simulink model "RL5_6kg_2021a_enc"  (R2021a)
settings: Solver=ode4  StartTime=0.0  StopTime=time(end)  FixedStep=0.001  RelTol=1e-6
model workspace: external: MATLAB File robot_6kg_v4_EXa5_DataFile.m (data not in the file)
values from neighbouring files (symbols this model uses):
  hI4 = I4wg + I4uch    [RL5_6kg_Dynamic_Param.m]
  hI5 = I5uch + I5ws    [RL5_6kg_Dynamic_Param.m]
  I4g = k4^2*Ig4    [RL5_6kg_Dynamic_Param.m]
  IAB = (Im + IA + IB)    [Basic_3DoF_Delta_Dynamic_Param.m]    (also in RL5_6kg_Dynamic_Param.m)
  lB = l1*(rho1*m1 + me)    [Basic_3DoF_Delta_Dynamic_Param.m]    (also in RL5_6kg_Dynamic_Param.m)
  m4 = 0    [Basic_3DoF_Delta_Dynamic_Param.m]    (also in RL5_6kg_Dynamic_Param.m = Inertias.Solid(10).mass)
  m5 = 0    [Basic_3DoF_Delta_Dynamic_Param.m]    (also in RL5_6kg_Dynamic_Param.m = Inertias.Solid(11).mass)
  m6l = 0    [Basic_3DoF_Delta_Dynamic_Param.m]    (also in RL5_6kg_Dynamic_Param.m = mls_a4 + mls_a5)
  m6u = 0    [Basic_3DoF_Delta_Dynamic_Param.m]    (also in RL5_6kg_Dynamic_Param.m = mus_a4 + mus_a5)
  mD = m3 + 3*m2 + 3*me    [Basic_3DoF_Delta_Dynamic_Param.m]    (also in RL5_6kg_Dynamic_Param.m = m3 + 3*m2 + 3*me + mls_a4_spi + mls_a5_spi + mls_a5_worm)
  rho2 = Sro2    [Basic_3DoF_Delta_Dynamic_Param.m]    (also in RL5_6kg_Dynamic_Param.m)
  rho6l = Sro6l    [RL5_6kg_Dynamic_Param.m]
  rho6u = Sro6u    [RL5_6kg_Dynamic_Param.m]
  tI4 = I4us + I4ls + I4ucr    [RL5_6kg_Dynamic_Param.m]
  tI5 = I5us + I5ls + I5ucr    [RL5_6kg_Dynamic_Param.m]
libraries: eeGeneralControl x5, simulink x5
settings Model: Creator=SUSTRVOJ  LastModifiedBy=alikoc
settings SolverCC: AlgebraicLoopSolver=TrustRegion
settings DataIOCC: SaveOutput=off  SignalLogging=off  DSMLogging=off  SaveTime=off  ReturnWorkspaceOutputs=off
settings DebuggingCC: SFMachineParentedDataDiag=warning
settings DiagnosticsConfigSet: SimMechanicsJointTargetOverSpecification=warning
settings ExplorerConfigSet: InternalSimMechanicsExplorerSettings="<ExplorerConfiguration><canonicalview>default</canonicalview><AnimationSetting><BasePlaybackSpeed>1.0</BasePlaybackSpeed><PlaybackSpeedFactor>1.0</PlaybackSpeedFactor></AnimationSetting><TilePanel><TileInfo><Tiles Columns=\"1\" Count=\"1\" Rows=\"1\"><Column Weight=\"1\"/><Row Weight=\"1\"/><Tile Height=\"1\" Width=\"1\" X=\"0\" Y=\"0\"/></Tiles></TileInfo><SceneInfo><SceneViewer><BGColor><R>0.60000002384185791</R><G>0.60000002384185791</G><B>0.60000002384185791</B></BGColor><Camera><DoPerspective>off</DoPerspective><Position><X>0.135215272225856747</X><Y>-1.20095496527992429</Y><Z>-0.491222676043407747</Z></Position><Center><X>0.135215272225856747</X><Y>5.5511151231257827e-17</Y><Z>-0.491222676043407747</Z></Center><Up><X>0</X><Y>-0</Y><Z>1</Z></Up><ViewLimDist>1</ViewLimDist><YLim>0.916798880077600797</YLim><XLim>1.0012025864974432</XLim></Camera></SceneViewer></SceneInfo></TilePanel><MechEditorPanel><Cameras/><GfxPanelCameraMap/><VideoCreator><PlaybackSpeedRatio>1.0</PlaybackSpeedRatio><FrameRate>30</FrameRate><VideoFormat>Motion JPEG AVI</VideoFormat><FrameSize>auto</FrameSize></VideoCreator></MechEditorPanel></ExplorerConfiguration>"

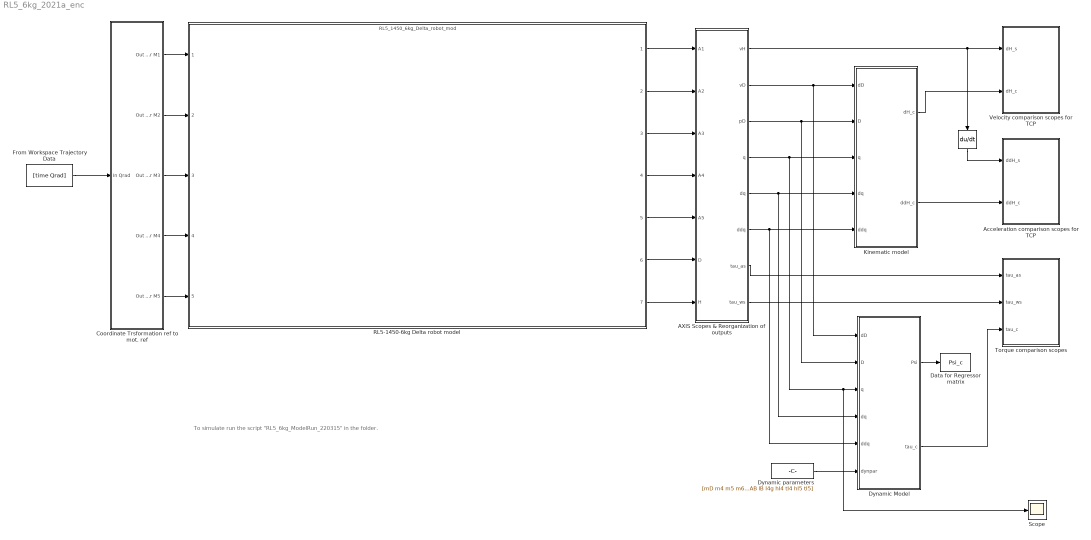
== system RL5_6kg_2021a_enc ==
  note: To simulate run the script "RL5_6kg_ModelRun_220315" in the folder.
  "   " : Derivative
  AXIS Scopes & Reorganization of outputs : Subsystem
  Acceleration comparison scopes for TCP : Subsystem
  Coordinate Trsformation ref to mot. ref : Subsystem
  Data for Regressor matrix : ToWorkspace  VariableName=Psi_c  SaveFormat=Structure With Time  SampleTime=-1
  Dynamic parameters : Constant  Value=[mD m4 m5 m6u m6l rho6u rho6l rho2 IAB lB I4g hI4 tI4 hI5 tI5]
  Dynamic Model : MATLAB Function  TreatAsAtomicUnit=on
  From Workspace Trajectory Data : FromWorkspace  VariableName=[time Qrad]  SampleTime=1e-3
  Kinematic model : MATLAB Function  TreatAsAtomicUnit=on
  RL5-1450-6kg Delta robot model : ModelReference  ModelNameDialog=RL5_1450_6kg_Delta_robot_mod.slxp  ModelReferenceVersion=1.1  CopyOfModelProtected=on
  Scope : Scope
  Torque comparison scopes : Subsystem
  Velocity comparison scopes for TCP : Subsystem
  wires:
  From Workspace Trajectory Data/1 -> Coordinate Trsformation ref to mot. ref/1(In Qrad)
  Coordinate Trsformation ref to mot. ref/1(Out rotor M1) -> RL5-1450-6kg Delta robot model/1
  Coordinate Trsformation ref to mot. ref/2(Out rotor M2) -> RL5-1450-6kg Delta robot model/2
  Coordinate Trsformation ref to mot. ref/3(Out rotor M3) -> RL5-1450-6kg Delta robot model/3
  Coordinate Trsformation ref to mot. ref/4(Out rotor M4) -> RL5-1450-6kg Delta robot model/4
  Coordinate Trsformation ref to mot. ref/5(Out rotor M5) -> RL5-1450-6kg Delta robot model/5
  RL5-1450-6kg Delta robot model/7 -> AXIS Scopes & Reorganization of outputs/7(H)
  RL5-1450-6kg Delta robot model/6 -> AXIS Scopes & Reorganization of outputs/6(D)
  RL5-1450-6kg Delta robot model/5 -> AXIS Scopes & Reorganization of outputs/5(A5)
  RL5-1450-6kg Delta robot model/4 -> AXIS Scopes & Reorganization of outputs/4(A4)
  RL5-1450-6kg Delta robot model/3 -> AXIS Scopes & Reorganization of outputs/3(A3)
  RL5-1450-6kg Delta robot model/2 -> AXIS Scopes & Reorganization of outputs/2(A2)
  RL5-1450-6kg Delta robot model/1 -> AXIS Scopes & Reorganization of outputs/1(A1)
  Dynamic Model/2(tau_c) -> Torque comparison scopes/3(tau_c)
  Dynamic parameters/1 -> Dynamic Model/6(dynpar)
  Kinematic model/1(dH_c) -> Velocity comparison scopes for TCP/2(dH_c)
  AXIS Scopes & Reorganization of outputs/1(vH) -> Velocity comparison scopes for TCP/1(dH_s), "   "/1
  Dynamic Model/1(Psi) -> Data for Regressor matrix/1
  Kinematic model/2(ddH_c) -> Acceleration comparison scopes for TCP/2(ddH_c)
  "   "/1 -> Acceleration comparison scopes for TCP/1(ddH_s)
  AXIS Scopes & Reorganization of outputs/3(pD) -> Kinematic model/2(D), Dynamic Model/2(D)
  AXIS Scopes & Reorganization of outputs/4(q) -> Kinematic model/3(q), Scope/1, Dynamic Model/3(q)
  AXIS Scopes & Reorganization of outputs/5(dq) -> Kinematic model/4(dq), Dynamic Model/4(dq)
  AXIS Scopes & Reorganization of outputs/6(ddq) -> Kinematic model/5(ddq), Dynamic Model/5(ddq)
  AXIS Scopes & Reorganization of outputs/7(tau_as) -> Torque comparison scopes/1(tau_as)
  AXIS Scopes & Reorganization of outputs/8(tau_ws) -> Torque comparison scopes/2(tau_ws)
  AXIS Scopes & Reorganization of outputs/2(vD) -> Kinematic model/1(dD), Dynamic Model/1(dD)

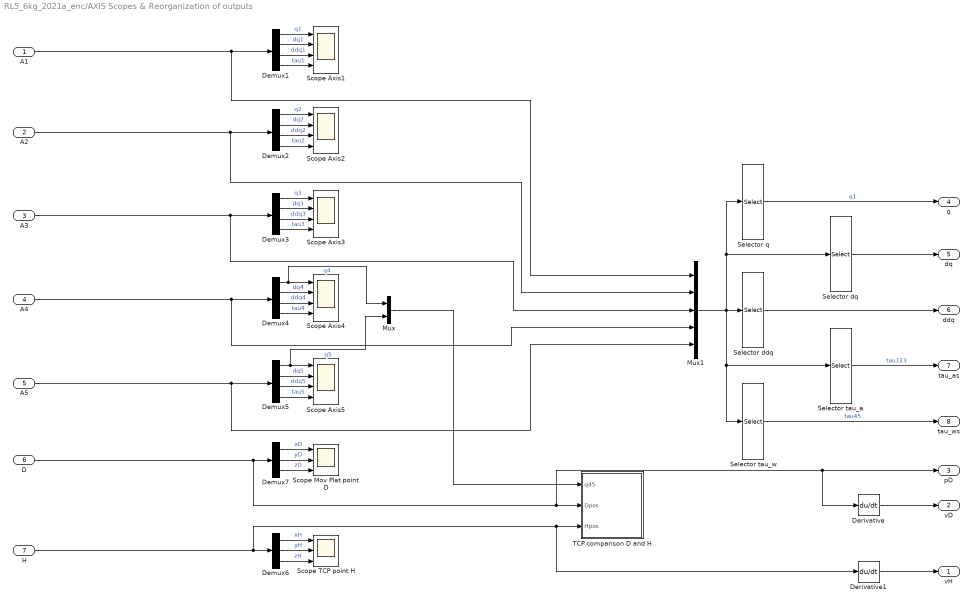
== system RL5_6kg_2021a_enc/AXIS Scopes & Reorganization of outputs ==
  A1 : Inport
  A2 : Inport  Port=2
  A3 : Inport  Port=3
  A4 : Inport  Port=4
  A5 : Inport  Port=5
  D : Inport  Port=6
  H : Inport  Port=7
  Demux{1..5} (5 alike) : Demux
  Demux6 : Demux  Outputs=3
  Demux7 : Demux  Outputs=3
  Derivative : Derivative
  Derivative1 : Derivative
  Mux : Mux  Inputs=2
  Mux1 : Mux  Inputs=5
  Scope Axis{1..5} (5 alike) : Scope  NumInputPorts=4
  Scope Mov Plat point D : Scope  NumInputPorts=3
  Scope TCP point H : Scope  NumInputPorts=3
  Selector ddq : Selector  InputPortWidth=20  IndexOptions=Index vector (dialog)  Indices=[3 7 11 15 19]  OutputSizes=1
  Selector dq : Selector  InputPortWidth=20  IndexOptions=Index vector (dialog)  Indices=[2 6 10 14 18]  OutputSizes=1
  Selector q : Selector  InputPortWidth=20  IndexOptions=Index vector (dialog)  Indices=[1 5 9 13 17]  OutputSizes=1
  Selector tau_a : Selector  InputPortWidth=20  IndexOptions=Index vector (dialog)  Indices=[4 8 12]  OutputSizes=1
  Selector tau_w : Selector  InputPortWidth=20  IndexOptions=Index vector (dialog)  Indices=[16 20]  OutputSizes=1
  TCP comparison D and H : Subsystem
  vH : Outport
  vD : Outport  Port=2
  pD : Outport  Port=3
  q : Outport  Port=4
  dq : Outport  Port=5
  ddq : Outport  Port=6
  tau_as : Outport  Port=7
  tau_ws : Outport  Port=8
  wires:
  A4/1 -> Mux1/4, Demux4/1
  A1/1 -> Mux1/1, Demux1/1
  A5/1 -> Mux1/5, Demux5/1
  D/1 -> TCP comparison D and H/2(Dpos), Derivative/1, pD/1, Demux7/1
  Demux3/2 -> Scope Axis3/2  "dq3"
  Demux3/3 -> Scope Axis3/3  "ddq3"
  Demux7/1 -> Scope Mov Plat point D/1  "xD"
  Demux5/1 -> Mux/2, Scope Axis5/1  "q5"
  Demux7/3 -> Scope Mov Plat point D/3  "zD"
  Demux5/3 -> Scope Axis5/3  "ddq5"
  Demux4/4 -> Scope Axis4/4  "tau4"
  Demux3/4 -> Scope Axis3/4  "tau3"
  Demux2/1 -> Scope Axis2/1  "q2"
  Demux7/2 -> Scope Mov Plat point D/2  "yD"
  Demux3/1 -> Scope Axis3/1  "q3"
  Demux6/1 -> Scope TCP point H/1  "xH"
  A3/1 -> Mux1/3, Demux3/1
  Demux5/4 -> Scope Axis5/4  "tau5"
  Demux6/2 -> Scope TCP point H/2  "yH"
  Demux4/2 -> Scope Axis4/2  "dq4"
  Demux2/4 -> Scope Axis2/4  "tau2"
  Demux6/3 -> Scope TCP point H/3  "zH"
  Demux1/4 -> Scope Axis1/4  "tau1"
  Demux4/1 -> Mux/1, Scope Axis4/1  "q4"
  A2/1 -> Mux1/2, Demux2/1
  Demux2/2 -> Scope Axis2/2  "dq2"
  Demux4/3 -> Scope Axis4/3  "ddq4"
  Demux5/2 -> Scope Axis5/2  "dq5"
  Demux2/3 -> Scope Axis2/3  "ddq2"
  Mux/1 -> TCP comparison D and H/1(q45)
  Demux1/1 -> Scope Axis1/1  "q1"
  Demux1/3 -> Scope Axis1/3  "ddq1"
  Demux1/2 -> Scope Axis1/2  "dq1"
  Selector ddq/1 -> ddq/1
  Selector q/1 -> q/1  "q1"
  Mux1/1 -> Selector ddq/1, Selector dq/1, Selector q/1, Selector tau_a/1, Selector tau_w/1
  Selector dq/1 -> dq/1
  Selector tau_a/1 -> tau_as/1  "tau123"
  Selector tau_w/1 -> tau_ws/1  "tau45"
  Derivative/1 -> vD/1
  H/1 -> Derivative1/1, TCP comparison D and H/3(Hpos), Demux6/1
  Derivative1/1 -> vH/1

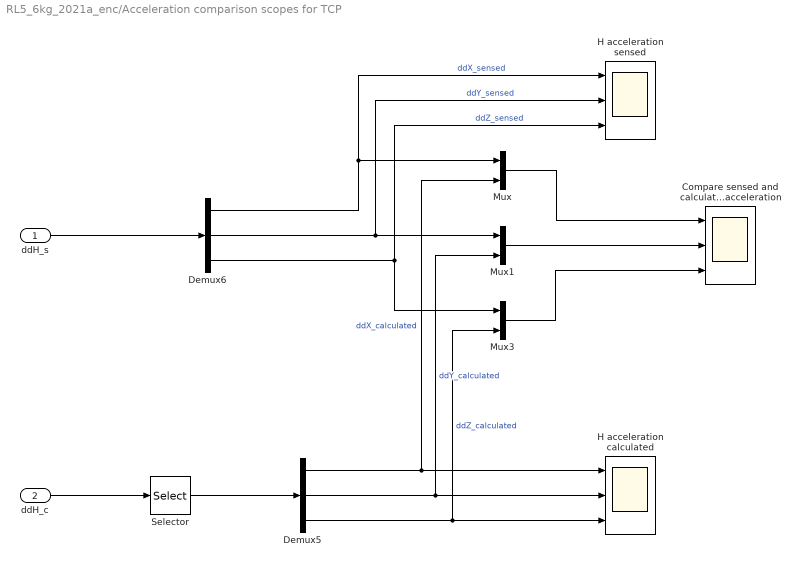
== system RL5_6kg_2021a_enc/Acceleration comparison scopes for TCP ==
  ddH_s : Inport
  ddH_c : Inport  Port=2
  Compare sensed and calculated H acceleration : Scope  NumInputPorts=3
  Demux5 : Demux  Outputs=3
  Demux6 : Demux  Outputs=3
  H acceleration calculated : Scope  NumInputPorts=3
  H acceleration sensed : Scope  NumInputPorts=3
  Mux : Mux  Inputs=2
  Mux1 : Mux  Inputs=2
  Mux3 : Mux  Inputs=2
  Selector : Selector  InputPortWidth=5  IndexOptions=Index vector (dialog)  Indices=[1 2 3]  OutputSizes=1
  wires:
  Demux6/3 -> H acceleration sensed/3, Mux3/1  "ddZ_sensed"
  Demux5/3 -> Mux3/2, H acceleration calculated/3  "ddZ_calculated"
  Demux5/2 -> H acceleration calculated/2, Mux1/2  "ddY_calculated"
  Demux6/2 -> H acceleration sensed/2, Mux1/1  "ddY_sensed"
  Demux6/1 -> H acceleration sensed/1, Mux/1  "ddX_sensed"
  ddH_s/1 -> Demux6/1
  Demux5/1 -> H acceleration calculated/1, Mux/2  "ddX_calculated"
  Mux1/1 -> Compare sensed and calculated H acceleration/2
  ddH_c/1 -> Selector/1
  Mux3/1 -> Compare sensed and calculated H acceleration/3
  Mux/1 -> Compare sensed and calculated H acceleration/1
  Selector/1 -> Demux5/1

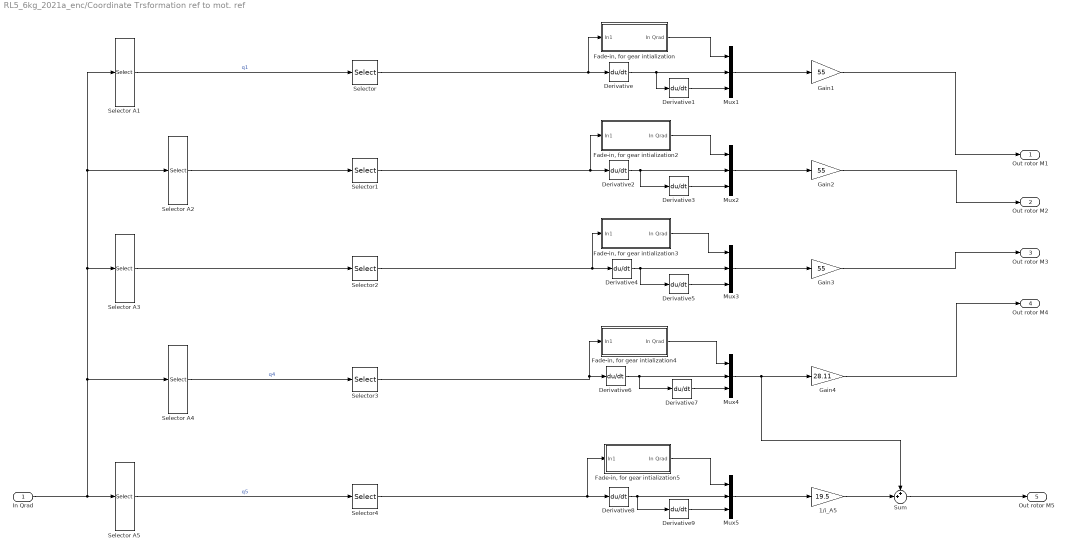
== system RL5_6kg_2021a_enc/Coordinate Trsformation ref to mot. ref ==
  In Qrad : Inport
  1/i_A5 : Gain  Gain=19.5
  Derivative{,1..9} (10 alike) : Derivative
  "Fade-in, for gear intialization" : Subsystem
  "Fade-in, for gear intialization2" : Subsystem
  "Fade-in, for gear intialization3" : Subsystem
  "Fade-in, for gear intialization4" : Subsystem
  "Fade-in, for gear intialization5" : Subsystem
  Gain1 : Gain  Gain=55
  Gain2 : Gain  Gain=55
  Gain3 : Gain  Gain=55
  Gain4 : Gain  Gain=28.11
  Mux{1..5} (5 alike) : Mux  Inputs=3
  Selector{,1..4} (5 alike) : Selector  InputPortWidth=3  IndexOptions=Index vector (dialog)  Indices=[1]  OutputSizes=1
  Selector A1 : Selector  InputPortWidth=15  IndexOptions=Index vector (dialog)  Indices=[1 6 11]  OutputSizes=1
  Selector A2 : Selector  InputPortWidth=15  IndexOptions=Index vector (dialog)  Indices=[2 7 12]  OutputSizes=1
  Selector A3 : Selector  InputPortWidth=15  IndexOptions=Index vector (dialog)  Indices=[3 8 13]  OutputSizes=1
  Selector A4 : Selector  InputPortWidth=15  IndexOptions=Index vector (dialog)  Indices=[4 9 14]  OutputSizes=1
  Selector A5 : Selector  InputPortWidth=15  IndexOptions=Index vector (dialog)  Indices=[5 10 15]  OutputSizes=1
  Sum : Sum  Inputs=++|
  Out rotor M1 : Outport
  Out rotor M2 : Outport  Port=2
  Out rotor M3 : Outport  Port=3
  Out rotor M4 : Outport  Port=4
  Out rotor M5 : Outport  Port=5
  wires:
  In Qrad/1 -> Selector A1/1, Selector A2/1, Selector A3/1, Selector A4/1, Selector A5/1
  Gain1/1 -> Out rotor M1/1
  Gain2/1 -> Out rotor M2/1
  Gain3/1 -> Out rotor M3/1
  Gain4/1 -> Out rotor M4/1
  1/i_A5/1 -> Sum/2
  Sum/1 -> Out rotor M5/1
  Derivative1/1 -> Mux1/3
  Derivative/1 -> Mux1/2, Derivative1/1
  Selector A1/1 -> Selector/1  "q1"
  Mux1/1 -> Gain1/1
  Mux2/1 -> Gain2/1
  Mux3/1 -> Gain3/1
  Mux4/1 -> Gain4/1, Sum/1
  Mux5/1 -> 1/i_A5/1
  Derivative3/1 -> Mux2/3
  Derivative2/1 -> Mux2/2, Derivative3/1
  Derivative5/1 -> Mux3/3
  Derivative4/1 -> Mux3/2, Derivative5/1
  Derivative6/1 -> Mux4/2, Derivative7/1
  Derivative7/1 -> Mux4/3
  Derivative8/1 -> Mux5/2, Derivative9/1
  Derivative9/1 -> Mux5/3
  Selector A4/1 -> Selector3/1  "q4"
  Selector A5/1 -> Selector4/1  "q5"
  Selector4/1 -> Derivative8/1, "Fade-in, for gear intialization5"/1(In1)
  Selector3/1 -> Derivative6/1, "Fade-in, for gear intialization4"/1(In1)
  Selector2/1 -> "Fade-in, for gear intialization3"/1(In1), Derivative4/1
  Selector1/1 -> "Fade-in, for gear intialization2"/1(In1), Derivative2/1
  Selector/1 -> "Fade-in, for gear intialization"/1(In1), Derivative/1
  Selector A3/1 -> Selector2/1
  "Fade-in, for gear intialization"/1(In Qrad) -> Mux1/1
  Selector A2/1 -> Selector1/1
  "Fade-in, for gear intialization4"/1(In Qrad) -> Mux4/1
  "Fade-in, for gear intialization5"/1(In Qrad) -> Mux5/1
  "Fade-in, for gear intialization2"/1(In Qrad) -> Mux2/1
  "Fade-in, for gear intialization3"/1(In Qrad) -> Mux3/1

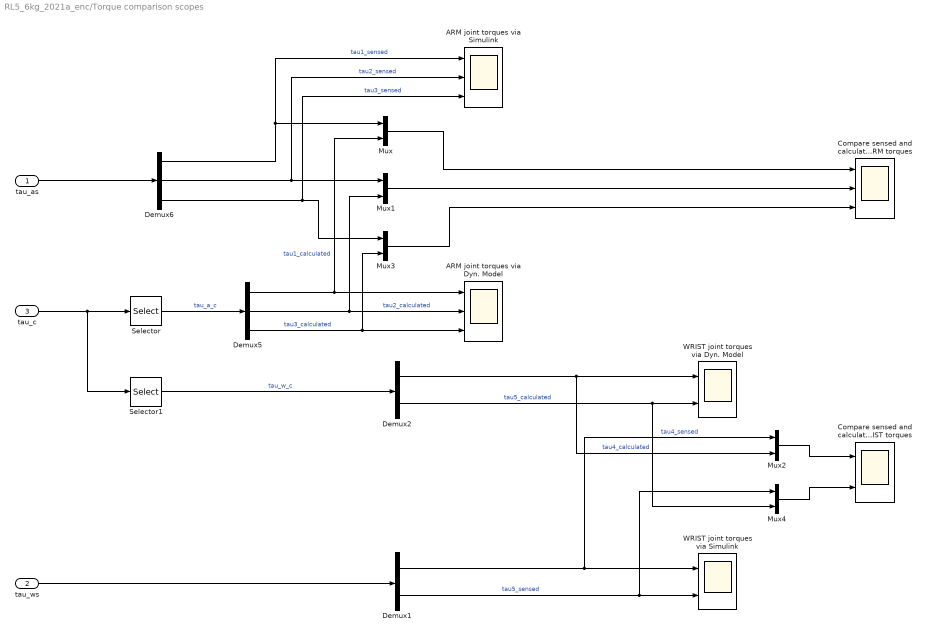
== system RL5_6kg_2021a_enc/Torque comparison scopes ==
  tau_as : Inport
  tau_ws : Inport  Port=2
  tau_c : Inport  Port=3
  "ARM joint torques via Dyn. Model " : Scope  NumInputPorts=3
  ARM joint torques via Simulink : Scope  NumInputPorts=3
  Compare sensed and calculated ARM torques : Scope  NumInputPorts=3
  Compare sensed and calculated WRIST torques : Scope  NumInputPorts=2
  Demux1 : Demux  Outputs=2
  Demux2 : Demux  Outputs=2
  Demux5 : Demux  Outputs=3
  Demux6 : Demux  Outputs=3
  Mux{,1..4} (5 alike) : Mux  Inputs=2
  Selector : Selector  InputPortWidth=5  IndexOptions=Index vector (dialog)  Indices=[1 2 3]  OutputSizes=1
  Selector1 : Selector  InputPortWidth=5  IndexOptions=Index vector (dialog)  Indices=[4 5]  OutputSizes=1
  WRIST joint torques via Dyn. Model : Scope  NumInputPorts=2
  WRIST joint torques via Simulink : Scope  NumInputPorts=2
  wires:
  Mux4/1 -> Compare sensed and calculated WRIST torques/2
  Mux2/1 -> Compare sensed and calculated WRIST torques/1
  Demux2/1 -> WRIST joint torques via Dyn. Model/1, Mux2/2  "tau4_calculated"
  Selector1/1 -> Demux2/1  "tau_w_c"
  Demux1/1 -> Mux2/1, WRIST joint torques via Simulink/1  "tau4_sensed"
  Demux1/2 -> WRIST joint torques via Simulink/2, Mux4/1  "tau5_sensed"
  tau_ws/1 -> Demux1/1
  Selector/1 -> Demux5/1  "tau_a_c"
  Mux/1 -> Compare sensed and calculated ARM torques/1
  Mux3/1 -> Compare sensed and calculated ARM torques/3
  tau_c/1 -> Selector/1, Selector1/1
  Mux1/1 -> Compare sensed and calculated ARM torques/2
  Demux5/1 -> Mux/2, "ARM joint torques via Dyn. Model "/1  "tau1_calculated"
  tau_as/1 -> Demux6/1
  Demux6/1 -> Mux/1, ARM joint torques via Simulink/1  "tau1_sensed"
  Demux6/2 -> Mux1/1, ARM joint torques via Simulink/2  "tau2_sensed"
  Demux5/2 -> Mux1/2, "ARM joint torques via Dyn. Model "/2  "tau2_calculated"
  Demux5/3 -> "ARM joint torques via Dyn. Model "/3, Mux3/2  "tau3_calculated"
  Demux6/3 -> Mux3/1, ARM joint torques via Simulink/3  "tau3_sensed"
  Demux2/2 -> Mux4/2, WRIST joint torques via Dyn. Model/2  "tau5_calculated"

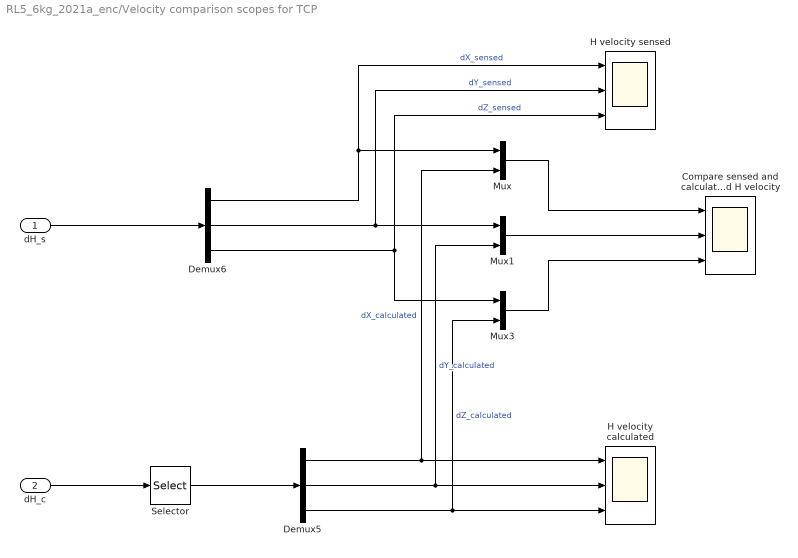
== system RL5_6kg_2021a_enc/Velocity comparison scopes for TCP ==
  dH_s : Inport
  dH_c : Inport  Port=2
  Compare sensed and calculated H velocity : Scope  NumInputPorts=3
  Demux5 : Demux  Outputs=3
  Demux6 : Demux  Outputs=3
  H velocity calculated : Scope  NumInputPorts=3
  H velocity sensed : Scope  NumInputPorts=3
  Mux : Mux  Inputs=2
  Mux1 : Mux  Inputs=2
  Mux3 : Mux  Inputs=2
  Selector : Selector  InputPortWidth=5  IndexOptions=Index vector (dialog)  Indices=[1 2 3]  OutputSizes=1
  wires:
  Selector/1 -> Demux5/1
  Mux/1 -> Compare sensed and calculated H velocity/1
  Mux3/1 -> Compare sensed and calculated H velocity/3
  dH_c/1 -> Selector/1
  Mux1/1 -> Compare sensed and calculated H velocity/2
  Demux5/1 -> Mux/2, H velocity calculated/1  "dX_calculated"
  dH_s/1 -> Demux6/1
  Demux6/1 -> Mux/1, H velocity sensed/1  "dX_sensed"
  Demux6/2 -> Mux1/1, H velocity sensed/2  "dY_sensed"
  Demux5/2 -> Mux1/2, H velocity calculated/2  "dY_calculated"
  Demux5/3 -> H velocity calculated/3, Mux3/2  "dZ_calculated"
  Demux6/3 -> Mux3/1, H velocity sensed/3  "dZ_sensed"

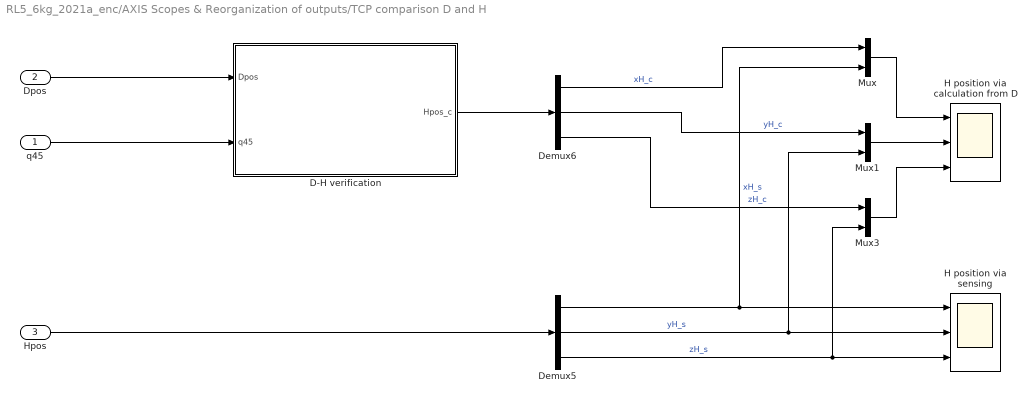
== system RL5_6kg_2021a_enc/AXIS Scopes & Reorganization of outputs/TCP comparison D and H ==
  q45 : Inport
  Dpos : Inport  Port=2
  Hpos : Inport  Port=3
  D-H verification : MATLAB Function  TreatAsAtomicUnit=on
  Demux5 : Demux  Outputs=3
  Demux6 : Demux  Outputs=3
  "H position via sensing " : Scope  NumInputPorts=3
  H position via calculation from D : Scope  NumInputPorts=3
  Mux : Mux  Inputs=2
  Mux1 : Mux  Inputs=2
  Mux3 : Mux  Inputs=2
  wires:
  Hpos/1 -> Demux5/1
  Demux5/2 -> "H position via sensing "/2, Mux1/2  "yH_s"
  Demux6/1 -> Mux/1  "xH_c"
  Demux5/1 -> "H position via sensing "/1, Mux/2  "xH_s"
  Demux6/2 -> Mux1/1  "yH_c"
  Mux1/1 -> H position via calculation from D/2
  Demux5/3 -> "H position via sensing "/3, Mux3/2  "zH_s"
  Demux6/3 -> Mux3/1  "zH_c"
  Mux/1 -> H position via calculation from D/1
  Mux3/1 -> H position via calculation from D/3
  q45/1 -> D-H verification/2(q45)
  Dpos/1 -> D-H verification/1(Dpos)
  D-H verification/1(Hpos_c) -> Demux6/1

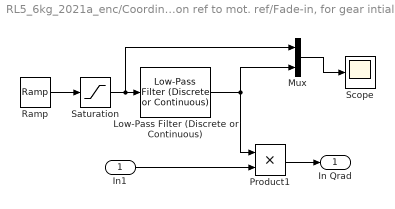
== system RL5_6kg_2021a_enc/Coordinate Trsformation ref to mot. ref/Fade-in, for gear intialization ==
  In1 : Inport
  Low-Pass Filter (Discrete or Continuous) : eeGeneralControl/Low-Pass Filter (Discrete or Continuous)  K=1  T=0.05  B=inf  A=-inf  init_option=Inherited from block input  x0=0  Ts=-1
  Mux : Mux  Inputs=2
  Product1 : Product
  Ramp : simulink/Sources/Ramp  slope=10  start=0.01  InitialOutput=0
  Saturation : Saturate  UpperLimit=1  LowerLimit=0
  Scope : Scope
  In Qrad : Outport
  wires:
  Mux/1 -> Scope/1
  Low-Pass Filter (Discrete or Continuous)/1 -> Product1/1, Mux/2
  Saturation/1 -> Low-Pass Filter (Discrete or Continuous)/1, Mux/1
  Product1/1 -> In Qrad/1
  In1/1 -> Product1/2
  Ramp/1 -> Saturation/1

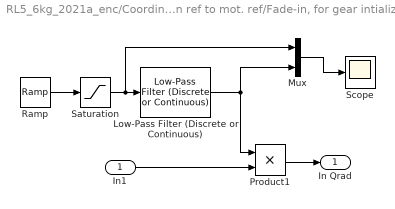
== system RL5_6kg_2021a_enc/Coordinate Trsformation ref to mot. ref/Fade-in, for gear intialization2 ==
  In1 : Inport
  Low-Pass Filter (Discrete or Continuous) : eeGeneralControl/Low-Pass Filter (Discrete or Continuous)  K=1  T=0.05  B=inf  A=-inf  init_option=Inherited from block input  x0=0  Ts=-1
  Mux : Mux  Inputs=2
  Product1 : Product
  Ramp : simulink/Sources/Ramp  slope=10  start=0.01  InitialOutput=0
  Saturation : Saturate  UpperLimit=1  LowerLimit=0
  Scope : Scope
  In Qrad : Outport
  wires:
  Ramp/1 -> Saturation/1
  In1/1 -> Product1/2
  Product1/1 -> In Qrad/1
  Saturation/1 -> Mux/1, Low-Pass Filter (Discrete or Continuous)/1
  Low-Pass Filter (Discrete or Continuous)/1 -> Mux/2, Product1/1
  Mux/1 -> Scope/1

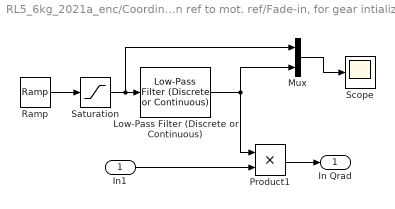
== system RL5_6kg_2021a_enc/Coordinate Trsformation ref to mot. ref/Fade-in, for gear intialization3 ==
  In1 : Inport
  Low-Pass Filter (Discrete or Continuous) : eeGeneralControl/Low-Pass Filter (Discrete or Continuous)  K=1  T=0.05  B=inf  A=-inf  init_option=Inherited from block input  x0=0  Ts=-1
  Mux : Mux  Inputs=2
  Product1 : Product
  Ramp : simulink/Sources/Ramp  slope=10  start=0.01  InitialOutput=0
  Saturation : Saturate  UpperLimit=1  LowerLimit=0
  Scope : Scope
  In Qrad : Outport
  wires:
  Mux/1 -> Scope/1
  Low-Pass Filter (Discrete or Continuous)/1 -> Product1/1, Mux/2
  Saturation/1 -> Low-Pass Filter (Discrete or Continuous)/1, Mux/1
  Product1/1 -> In Qrad/1
  In1/1 -> Product1/2
  Ramp/1 -> Saturation/1

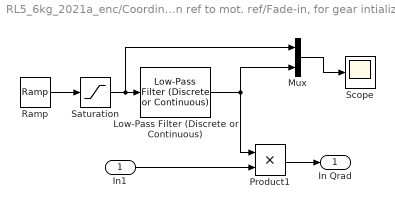
== system RL5_6kg_2021a_enc/Coordinate Trsformation ref to mot. ref/Fade-in, for gear intialization4 ==
  In1 : Inport
  Low-Pass Filter (Discrete or Continuous) : eeGeneralControl/Low-Pass Filter (Discrete or Continuous)  K=1  T=0.05  B=inf  A=-inf  init_option=Inherited from block input  x0=0  Ts=-1
  Mux : Mux  Inputs=2
  Product1 : Product
  Ramp : simulink/Sources/Ramp  slope=10  start=0.01  InitialOutput=0
  Saturation : Saturate  UpperLimit=1  LowerLimit=0
  Scope : Scope
  In Qrad : Outport
  wires:
  Ramp/1 -> Saturation/1
  In1/1 -> Product1/2
  Product1/1 -> In Qrad/1
  Saturation/1 -> Mux/1, Low-Pass Filter (Discrete or Continuous)/1
  Low-Pass Filter (Discrete or Continuous)/1 -> Mux/2, Product1/1
  Mux/1 -> Scope/1

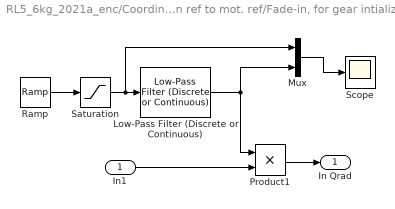
== system RL5_6kg_2021a_enc/Coordinate Trsformation ref to mot. ref/Fade-in, for gear intialization5 ==
  In1 : Inport
  Low-Pass Filter (Discrete or Continuous) : eeGeneralControl/Low-Pass Filter (Discrete or Continuous)  K=1  T=0.05  B=inf  A=-inf  init_option=Inherited from block input  x0=0  Ts=-1
  Mux : Mux  Inputs=2
  Product1 : Product
  Ramp : simulink/Sources/Ramp  slope=10  start=0.01  InitialOutput=0
  Saturation : Saturate  UpperLimit=1  LowerLimit=0
  Scope : Scope
  In Qrad : Outport
  wires:
  Mux/1 -> Scope/1
  Low-Pass Filter (Discrete or Continuous)/1 -> Product1/1, Mux/2
  Saturation/1 -> Low-Pass Filter (Discrete or Continuous)/1, Mux/1
  Product1/1 -> In Qrad/1
  In1/1 -> Product1/2
  Ramp/1 -> Saturation/1

== matlab function RL5_6kg_2021a_enc/Dynamic Model ==
  data: Psi output; dD input; D input; q input; dq input; ddq input; dynpar input; tau_c output
function [Psi,tau_c] = dyn(dD,D,q,dq,ddq,dynpar)
% This function block represents mathematical DYNAMIC MODEL 

q0 = 5.327998*pi/180;   % [rad], 5.327998° ~ q0*pi/180 rad, angle( axis_i & line(A_i,B_i) )
r0 =  0.330;            % [m], radius of circumscribed circle of equilat. basic frame triangle
l1 =  0.420;            % [m], lengths of upper arms
% l2 =  1.055;          % [m], lengths of forearms, not used
r3 =  0.125;            % [m], radius of circumscribed circle of equilat. mov. platform trngl.
r4 =  0.0632;           % [m], radius of wrist arm offset, distance from point E to F
r4m = 0.0424798;        % [m], radius of wrist arm CoG point offset,distance from point E to \bar{F} 
% h4 =  0.132;          % [m], perpendicular distance from point D to E (h4m = h4), not used
% r5 =  0.135;          % [m], radius of swivel arm (distance A5-axis vs. Tool Center Point (TCP)), not used
r5m = 0.1225 - 0.0432725;       % distance from F to the CoG of the swivel arm; translation in Z = 0.1225, Inertias.Solid(11).CoM(3)=0.0432725. 
dr =  r0 - r3;                  % [m], useful simplifying constant

% Actuated joint positions
q1 = q(1) - q0; q2 = q(2) - q0;  q3 = q(3) - q0;  q4 = q(4);  q5 = q(5);

% Actuated joint velocities
dq1 = dq(1);  dq2 = dq(2);  dq3 = dq(3);  dq4 = dq(4);  dq5 = dq(5);

% Actuated joint accelerations
ddq1 = ddq(1);  ddq2 = ddq(2);  ddq3 = ddq(3);  ddq4 = ddq(4);  ddq5 = ddq(5);

% Point D positions
xD = D(1);  yD = D(2);  zD = D(3); 

% Point D velocities
dxD = dD(1);  dyD = dD(2);  dzD = dD(3);

%% Dynamic model mass parameters
g = 9.80665; % [m]/s^2, gravity

mD = dynpar(1);     % Constant total mass at movable platform level (point D)

m4 = dynpar(2);     % mass of the wrist arm
m5 = dynpar(3);     % mass of the swivel arm

%% Jacobian matrices J_D, J_q, J_\mathcal{D} and their derivatives and inverses

[Jd,Jq] = Jcq(xD,yD,zD,dr,l1,q1,q2,q3);             % Eq (17) in the paper: Jd = J_D, Jq = J_q 
Jqd = Jd\Jq; iJqd = Jq\Jd;                          % Eq (18) in the paper: Jqd = J_qD, iJqd = J_qD^{-1}

JD = [Jqd, zeros(3,2); zeros(2,3), eye(2)];         % Eq (19) in the paper: JD = J_\mathcal{D}
% iJD = [iJqd, zeros(3,2) ; zeros(2,3), eye(2)];      % Eq (19) in the paper: iJD = J_\mathcal{D}^{-1}

[dJc,dJq] = dJcq(xD,yD,zD,dxD,dyD,dzD,dr,l1,q1,q2,q3,dq1,dq2,dq3); 
dJqd = Jd\(dJq-dJc*Jqd);                            % Eq (22) in the paper: derivative of J_qD

dJD = [dJqd, zeros(3,2) ; zeros(2,3), zeros(2)];    % derivative of J_\mathcal{D}

Jqd_4 = [Jqd, zeros(3,1) ; zeros(1,3), 1];          % One of the matrix in Eq. (25)

%% Jacobians and their derivatives for CoG of swivel arm (A5)

[c11,c21,c31,c12,c22,c32] = f_cii(r4,r5m,q4,q5);    
Jsc = [c11, c12 ; c21, c22 ; c31, c32]; 
iJDH = [eye(3), Jsc ; zeros(2,3), eye(2)];          % Eq (15) in the paper: iJDH = J_\mathcal{DH}^{-1}

JH = iJDH\JD;                                       % Eq (26) with (19) in the paper: J_\mathcal{H} = J_\mathcal{DH}^{-1}*J_\mathcal{D}

[dc11,dc21,dc31,dc12,dc22,dc32] = f_deriv_cii(r4,r5m,q4,q5,dq4,dq5); 
dJsc = [dc11, dc12 ; dc21, dc22 ; dc31, dc32]; 
diJDH = [zeros(3), dJsc ; zeros(2,3), zeros(2)];    % derivative of J_\mathcal{DH}

dJH = (iJDH\(dJD - diJDH*JH));                      % derivative of J_\mathcal{H}

%% Jacobians and their derivatives for CoG of wrist arm (A4)

[c11F,c21F,c31F,dc11F,dc21F,dc31F] = f_d_ciiF(r4m,q4,dq4);
JscF = [c11F ; c21F ; c31F];                    
JsF = [eye(3), JscF ; zeros(1,3), 1];

JF = [ JsF\Jqd_4 , zeros(4,1) ; zeros(1,5) ] ;       % Eq (25) with (19) in the paper: JF = J_\mathcal{F}

iJDF = [JsF, zeros(4,1) ; zeros(1,5)]; 
dJscF = [dc11F, 0 ; dc21F, 0 ; dc31F, 0];           
diJDF = [zeros(3), dJscF ; zeros(2,3), zeros(2)];    

dJF = (iJDF\(dJD - diJDF*JF));                       % derivative of J_\mathcal{F} 

%% Dynamical model of the parallel part (A1-A2-A3): Equation of Motion: Eq. (37) with (48)

ld = sqrt(xD^2+yD^2);                   % distance of point D inn XY plane from point O

m6u = dynpar(4);    m6l = dynpar(5);    % total mass of upper and lower tel. shaft parts 
rho6u = dynpar(6);  rho6l = dynpar(7);  % mass distribution ratios for upper and lower tel. shaft parts 

m2 = 1.05;
rho2 = dynpar(8);                       % mass distribution ratio for upper arms 

mD =  mD - ( rho2*m2*(cos(q1)+cos(q2)+cos(q3)) );    % the mass of the movable platform with trajectoryy-dependent contribution of forearm masses
mDs = (rho6u*ld*m6u + (1-ld)*rho6l*m6l);             % the contribution of shaft masses to the movable platform 

IAB = dynpar(9);                                     % fixed inertia values of each upper arm excluding the effect of m2
IAB = diag([IAB + l1^2*rho2*cos(q1)*m2, IAB + l1^2*rho2*cos(q2)*m2, IAB + l1^2*rho2*cos(q3)*m2, 0, 0]); % inertia matrix for upper arms 

I_35 = [eye(3), zeros(3,2)];
Ma = I_35*( IAB + mD*(JD'*JD) + m4*(JF'*JF) + m5*(JH'*JH) );    % Eq. (48) in the paper: Inertial matrix for the parallel part
Ca = I_35*( mD*JD'*dJD + m4*JF'*dJF + m5*JH'*dJH ) ;            % Eq. (48) in the paper: Coriolis & centrifugal matrix for the parallel part

lBnum = dynpar(10);     
Ga = I_35*diag([lBnum + l1*rho2*cos(q1)*m2, lBnum + l1*rho2*cos(q2)*m2, lBnum + l1*rho2*cos(q3)*m2, 0, 0])*g*[cos(q1); cos(q2); cos(q3); 0; 0] ...
   - I_35*( (mD+mDs)*JD'+m4*JF'+m5*JH' )*[0; 0; -g; 0; 0] ;     % Eq. (48) with (45) in the paper: Gravitational matrix for the parallel part

tau_a = Ma*ddq + Ca*dq + Ga ;                                   % Torque vector of the actuated upper arms 

%% Collecting data for the regressor matrix (61) of the regression model from the sampled values of (59)
% This part is used only for the first simulation to collect data for mass
% distribution ratio estimation, can be commentted out after estimation
Sig10 = ddq1; 
Sig14 = g*JF(3,1) + dq1*(dJF(1,1)*JF(1,1) + dJF(2,1)*JF(2,1) + dJF(3,1)*JF(3,1) + dJF(4,1)*JF(4,1)) + dq2*(dJF(1,2)*JF(1,1) + dJF(2,2)*JF(2,1) + dJF(3,2)*JF(3,1) + dJF(4,2)*JF(4,1)) + dq3*(dJF(1,3)*JF(1,1) + dJF(2,3)*JF(2,1) + dJF(3,3)*JF(3,1) + dJF(4,3)*JF(4,1)) + dq4*(dJF(1,4)*JF(1,1) + dJF(2,4)*JF(2,1) + dJF(3,4)*JF(3,1) + dJF(4,4)*JF(4,1)) + ddq1*(JF (1,1)^2 + JF (2,1)^2 + JF (3,1)^2 + JF (4,1)^2) + ddq2*(JF(1,1)*JF(1,2) + JF(2,1)*JF(2,2) + JF(3,1)*JF(3,2) + JF(4,1)*JF(4,2)) + ddq3*(JF(1,1)*JF(1,3) + JF(2,1)*JF(2,3) + JF(3,1)*JF(3,3) + JF(4,1)*JF(4,3)) + ddq4*(JF(1,1)*JF(1,4) + JF(2,1)*JF(2,4) + JF(3,1)*JF(3,4) + JF(4,1)*JF(4,4));
Sig15 = g*JH(3,1) + dq1*(dJH(1,1)*JH(1,1) + dJH(2,1)*JH(2,1) + dJH(3,1)*JH(3,1) + dJH(4,1)*JH(4,1) + dJH(5,1)*JH(5,1)) + dq2*(dJH(1,2)*JH(1,1) + dJH(2,2)*JH(2,1) + dJH(3,2)*JH(3,1) + dJH(4,2)*JH(4,1) + dJH(5,2)*JH(5,1)) + dq3*(dJH(1,3)*JH(1,1) + dJH(2,3)*JH(2,1) + dJH(3,3)*JH(3,1) + dJH(4,3)*JH(4,1) + dJH(5,3)*JH(5,1)) + dq4*(dJH(1,4)*JH(1,1) + dJH(2,4)*JH(2,1) + dJH(3,4)*JH(3,1) + dJH(4,4)*JH(4,1) + dJH(5,4)*JH(5,1)) + dq5*(dJH(1,5)*JH(1,1) + dJH(2,5)*JH(2,1) + dJH(3,5)*JH(3,1) + dJH(4,5)*JH(4,1) + dJH(5,5)*JH(5,1)) + ddq1*(JH (1,1)^2 + JH (2,1)^2 + JH (3,1)^2 + JH (4,1)^2 + JH (5,1)^2) + ddq2*(JH(1,1)*JH(1,2) + JH(2,1)*JH(2,2) + JH(3,1)*JH(3,2) + JH(4,1)*JH(4,2) + JH(5,1)*JH(5,2)) + ddq3*(JH(1,1)*JH(1,3) + JH(2,1)*JH(2,3) + JH(3,1)*JH(3,3) + JH(4,1)*JH(4,3) + JH(5,1)*JH(5,3)) + ddq4*(JH(1,1)*JH(1,4) + JH(2,1)*JH(2,4) + JH(3,1)*JH(3,4) + JH(4,1)*JH(4,4) + JH(5,1)*JH(5,4)) + ddq5*(JH(1,1)*JH(1,5) + JH(2,1)*JH(2,5) + JH(3,1)*JH(3,5) + JH(4,1)*JH(4,5) + JH(5,1)*JH(5,5));
Sig1D = g*JD(3,1) + dq1*(dJqd(1,1)*JD(1,1) + dJqd(2,1)*JD(2,1) + dJqd(3,1)*JD(3,1)) + dq2*(dJqd(1,2)*JD(1,1) + dJqd(2,2)*JD(2,1) + dJqd(3,2)*JD(3,1)) + dq3*(dJqd(1,3)*JD(1,1) + dJqd(2,3)*JD(2,1) + dJqd(3,3)*JD(3,1)) + ddq1*(JD (1,1)^2 + JD (2,1)^2 + JD (3,1)^2) + ddq2*(JD(1,1)*JD(1,2) + JD(2,1)*JD(2,2) + JD(3,1)*JD(3,2)) + ddq3*(JD(1,1)*JD(1,3) + JD(2,1)*JD(2,3) + JD(3,1)*JD(3,3));
Sig1Ds = g*JD(3,1);
%
Sig20 = ddq2; 
Sig24 = g*JF(3,2) + dq1*(dJF(1,1)*JF(1,2) + dJF(2,1)*JF(2,2) + dJF(3,1)*JF(3,2) + dJF(4,1)*JF(4,2)) + dq2*(dJF(1,2)*JF(1,2) + dJF(2,2)*JF(2,2) + dJF(3,2)*JF(3,2) + dJF(4,2)*JF(4,2)) + dq3*(dJF(1,3)*JF(1,2) + dJF(2,3)*JF(2,2) + dJF(3,3)*JF(3,2) + dJF(4,3)*JF(4,2)) + dq4*(dJF(1,4)*JF(1,2) + dJF(2,4)*JF(2,2) + dJF(3,4)*JF(3,2) + dJF(4,4)*JF(4,2)) + ddq1*(JF(1,1)*JF(1,2) + JF(2,1)*JF(2,2) + JF(3,1)*JF(3,2) + JF(4,1)*JF(4,2)) + ddq2*(JF (1,2)^2 + JF (2,2)^2 + JF (3,2)^2 + JF (4,2)^2) + ddq3*(JF(1,2)*JF(1,3) + JF(2,2)*JF(2,3) + JF(3,2)*JF(3,3) + JF(4,2)*JF(4,3)) + ddq4*(JF(1,2)*JF(1,4) + JF(2,2)*JF(2,4) + JF(3,2)*JF(3,4) + JF(4,2)*JF(4,4)); 
Sig25 = g*JH(3,2) + dq1*(dJH(1,1)*JH(1,2) + dJH(2,1)*JH(2,2) + dJH(3,1)*JH(3,2) + dJH(4,1)*JH(4,2) + dJH(5,1)*JH(5,2)) + dq2*(dJH(1,2)*JH(1,2) + dJH(2,2)*JH(2,2) + dJH(3,2)*JH(3,2) + dJH(4,2)*JH(4,2) + dJH(5,2)*JH(5,2)) + dq3*(dJH(1,3)*JH(1,2) + dJH(2,3)*JH(2,2) + dJH(3,3)*JH(3,2) + dJH(4,3)*JH(4,2) + dJH(5,3)*JH(5,2)) + dq4*(dJH(1,4)*JH(1,2) + dJH(2,4)*JH(2,2) + dJH(3,4)*JH(3,2) + dJH(4,4)*JH(4,2) + dJH(5,4)*JH(5,2)) + dq5*(dJH(1,5)*JH(1,2) + dJH(2,5)*JH(2,2) + dJH(3,5)*JH(3,2) + dJH(4,5)*JH(4,2) + dJH(5,5)*JH(5,2)) + ddq1*(JH(1,1)*JH(1,2) + JH(2,1)*JH(2,2) + JH(3,1)*JH(3,2) + JH(4,1)*JH(4,2) + JH(5,1)*JH(5,2)) + ddq2*(JH (1,2)^2 + JH (2,2)^2 + JH (3,2)^2 + JH (4,2)^2 + JH (5,2)^2) + ddq3*(JH(1,2)*JH(1,3) + JH(2,2)*JH(2,3) + JH(3,2)*JH(3,3) + JH(4,2)*JH(4,3) + JH(5,2)*JH(5,3)) + ddq4*(JH(1,2)*JH(1,4) + JH(2,2)*JH(2,4) + JH(3,2)*JH(3,4) + JH(4,2)*JH(4,4) + JH(5,2)*JH(5,4)) + ddq5*(JH(1,2)*JH(1,5) + JH(2,2)*JH(2,5) + JH(3,2)*JH(3,5) + JH(4,2)*JH(4,5) + JH(5,2)*JH(5,5)); 
Sig2D = g*JD(3,2) + dq1*(dJqd(1,1)*JD(1,2) + dJqd(2,1)*JD(2,2) + dJqd(3,1)*JD(3,2)) + dq2*(dJqd(1,2)*JD(1,2) + dJqd(2,2)*JD(2,2) + dJqd(3,2)*JD(3,2)) + dq3*(dJqd(1,3)*JD(1,2) + dJqd(2,3)*JD(2,2) + dJqd(3,3)*JD(3,2)) + ddq1*(JD(1,1)*JD(1,2) + JD(2,1)*JD(2,2) + JD(3,1)*JD(3,2)) + ddq2*(JD (1,2)^2 + JD (2,2)^2 + JD (3,2)^2) + ddq3*(JD(1,2)*JD(1,3) + JD(2,2)*JD(2,3) + JD(3,2)*JD(3,3)); 
Sig2Ds = g*JD(3,2);
%
Sig30 = ddq3; 
Sig34 = g*JF(3,3) + dq1*(dJF(1,1)*JF(1,3) + dJF(2,1)*JF(2,3) + dJF(3,1)*JF(3,3) + dJF(4,1)*JF(4,3)) + dq2*(dJF(1,2)*JF(1,3) + dJF(2,2)*JF(2,3) + dJF(3,2)*JF(3,3) + dJF(4,2)*JF(4,3)) + dq3*(dJF(1,3)*JF(1,3) + dJF(2,3)*JF(2,3) + dJF(3,3)*JF(3,3) + dJF(4,3)*JF(4,3)) + dq4*(dJF(1,4)*JF(1,3) + dJF(2,4)*JF(2,3) + dJF(3,4)*JF(3,3) + dJF(4,4)*JF(4,3)) + ddq1*(JF(1,1)*JF(1,3) + JF(2,1)*JF(2,3) + JF(3,1)*JF(3,3) + JF(4,1)*JF(4,3)) + ddq2*(JF(1,2)*JF(1,3) + JF(2,2)*JF(2,3) + JF(3,2)*JF(3,3) + JF(4,2)*JF(4,3)) + ddq3*(JF (1,3)^2 + JF (2,3)^2 + JF (3,3)^2 + JF (4,3)^2) + ddq4*(JF(1,3)*JF(1,4) + JF(2,3)*JF(2,4) + JF(3,3)*JF(3,4) + JF(4,3)*JF(4,4));
Sig35 = g*JH(3,3) + dq1*(dJH(1,1)*JH(1,3) + dJH(2,1)*JH(2,3) + dJH(3,1)*JH(3,3) + dJH(4,1)*JH(4,3) + dJH(5,1)*JH(5,3)) + dq2*(dJH(1,2)*JH(1,3) + dJH(2,2)*JH(2,3) + dJH(3,2)*JH(3,3) + dJH(4,2)*JH(4,3) + dJH(5,2)*JH(5,3)) + dq3*(dJH(1,3)*JH(1,3) + dJH(2,3)*JH(2,3) + dJH(3,3)*JH(3,3) + dJH(4,3)*JH(4,3) + dJH(5,3)*JH(5,3)) + dq4*(dJH(1,4)*JH(1,3) + dJH(2,4)*JH(2,3) + dJH(3,4)*JH(3,3) + dJH(4,4)*JH(4,3) + dJH(5,4)*JH(5,3)) + dq5*(dJH(1,5)*JH(1,3) + dJH(2,5)*JH(2,3) + dJH(3,5)*JH(3,3) + dJH(4,5)*JH(4,3) + dJH(5,5)*JH(5,3)) + ddq1*(JH(1,1)*JH(1,3) + JH(2,1)*JH(2,3) + JH(3,1)*JH(3,3) + JH(4,1)*JH(4,3) + JH(5,1)*JH(5,3)) + ddq2*(JH(1,2)*JH(1,3) + JH(2,2)*JH(2,3) + JH(3,2)*JH(3,3) + JH(4,2)*JH(4,3) + JH(5,2)*JH(5,3)) + ddq3*(JH (1,3)^2 + JH (2,3)^2 + JH (3,3)^2 + JH (4,3)^2 + JH (5,3)^2) + ddq4*(JH(1,3)*JH(1,4) + JH(2,3)*JH(2,4) + JH(3,3)*JH(3,4) + JH(4,3)*JH(4,4) + JH(5,3)*JH(5,4)) + ddq5*(JH(1,3)*JH(1,5) + JH(2,3)*JH(2,5) + JH(3,3)*JH(3,5) + JH(4,3)*JH(4,5) + JH(5,3)*JH(5,5));
Sig3D = g*JD(3,3)+dq1*(dJqd(1,1)*JD(1,3)+dJqd(2,1)*JD(2,3)+dJqd(3,1)*JD(3,3))+dq2*(dJqd(1,2)*JD(1,3)+dJqd(2,2)*JD(2,3)+dJqd(3,2)*JD(3,3))+dq3*(dJqd(1,3)*JD(1,3)+dJqd(2,3)*JD(2,3)+dJqd(3,3)*JD(3,3))+ddq1*(JD(1,1)*JD(1,3)+JD(2,1)*JD(2,3)+JD(3,1)*JD(3,3))+ddq2*(JD(1,2)*JD(1,3)+JD(2,2)*JD(2,3)+JD(3,2)*JD(3,3))+ddq3*(JD (1,3)^2+JD (2,3)^2+JD (3,3)^2); 
Sig3Ds = g*JD(3,3);
%
Psi = [ Sig10, Sig10*cos(q1), Sig14, Sig15, Sig1D, -Sig1D*(cos(q1)+cos(q2)+cos(q3)), Sig1Ds*ld, Sig1Ds, -Sig1Ds*ld, g*cos(q1), g*(cos(q1))^2 ; ...
        Sig20, Sig20*cos(q2), Sig24, Sig25, Sig2D, -Sig2D*(cos(q1)+cos(q2)+cos(q3)), Sig2Ds*ld, Sig2Ds, -Sig2Ds*ld, g*cos(q2), g*(cos(q2))^2 ; ...
        Sig30, Sig30*cos(q3), Sig34, Sig35, Sig3D, -Sig3D*(cos(q1)+cos(q2)+cos(q3)), Sig3Ds*ld, Sig3Ds, -Sig3Ds*ld, g*cos(q3), g*(cos(q3))^2 ] ;
    
%% Angular acceleration of the telescopic shafts A4 and A5 

zd = zD + 0.042;                        % The lower extremity of the shafts are 0.042 m higher in z-axis than point D
alpha = atan2(yD,xD);                   % Azimuth angle of the telescopic shafts 

eps = atan2(zd,sqrt(xD^2+yD^2));        % Elevation angle of the telescopic shafts 
teps = pi/2 + eps;                      % \tilde{\epsilon} Eq. (31) in the paper: Argument of the rotation matrix R_y in Eq. (30)

% Angular acceleration and velocity of the tel. shaft A4
ddtq4 = (cos(teps)*(-sin(teps)^2*sin(2*(alpha-q4))*dq4^2 + (cos(alpha-q4)^2+cos(teps)^2*sin(alpha-q4)^2)*ddq4))/(cos(alpha-q4)^2+ cos(teps)^2*sin(alpha-q4)^2)^2;

k5 = 19.5;                      % worm gear reduction ratio for A5
v5 = q4 + k5*q5;                % angular position of the input shaft for A5

dv5 = dq4 + k5*dq5;             % angular velocity of the input shaft for A5
ddv5 = ddq4 + k5*ddq5;          % angular acceleration of the input shaft for A5

% Angular acceleration and velocity of the tel. shaft A5
ddtq5 = (cos(teps)*(-sin(teps)^2*sin(2*(alpha-v5))*dv5^2 + (cos(alpha-v5)^2+cos(teps)^2*sin(alpha-v5)^2)*ddv5))/(cos(alpha-v5)^2+ cos(teps)^2*sin(alpha-v5)^2)^2;

%% Dynamical model of the serial part (A4-A5): Equation of Motion: Eq. (49) with (..)

I4g = dynpar(11) ;      % = k4^2*Ig4 -- Eq. (55)
hI4 = dynpar(12);       % = I4wg + I4uch -- Eq. (55)
tI4 = dynpar(13);       % = I4us + I4ls + I4ucr -- Eq. (55)

hI5 = dynpar(14);       % = I5uch + I5ws -- Eq. (52)
tI5 = dynpar(15);       % = I5us + I5ls + I5ucr -- Eq. (52)

Iw = [I4g + hI4, 0 ; hI5 , k5*hI5]; 
X1 = [zeros(2,3), [1, 0 ; 0 , 0]]; 
X2 = [zeros(2,3), [0, -1/k5 ; 0 , 1/k5]];
M4 = JF'*JF - JD'*JD ; 
M5 = JH'*JH - JD'*JD ;
Mw = [zeros(2,3), Iw] + [X1, X2]*[ m4*M4+m5*M5 ; m5*M5] ; % Eq. (57) in the paper: Inertial matrix for the serial part

C4 = JF'*dJF - JD'*dJD ; 
C5 = JH'*dJH - JD'*dJD ;
Cw = [X1, X2]*[ m4*C4+m5*C5 ; m5*C5] ;                    % Eq. (57) in the paper: Coriolis & centrifugal matrix for the serial part

Gw = [-r5m*m5*g*sin(q5)/19.5 ; r5m*m5*g*sin(q5)/19.5 ] ;  % Eq. (57) in the paper: Gravitational matrix for the serial part

tau_w = Mw*ddq + Cw*dq + Gw + [tI4*ddtq4 ; tI5*ddtq5] ;   % Eq. (49) in the paper: Torque vector to be applied to shafts drive joints

%% ALL ACTUATED JOINT TORQUE VECTORS

tau_c = [tau_a ; tau_w];                                  % Eq. (58) in the paper: Overall dynamic model of the robot

end

function [Jc,Jq] = Jcq(xD,yD,zD,dr,l1,q1,q2,q3)
Jc = [ 2*xD - 2*dr - 2*l1*cos(q1), 2*yD, 2*zD - 2*l1*sin(q1); ...
       dr + 2*xD + l1*cos(q2), 2*yD - 3^(1/2)*dr - 3^(1/2)*l1*cos(q2), 2*zD - 2*l1*sin(q2); ...
       dr + 2*xD + l1*cos(q3), 2*yD + 3^(1/2)*dr + 3^(1/2)*l1*cos(q3), 2*zD - 2*l1*sin(q3)];
Jq = [ 2*l1*(dr*sin(q1) + zD*cos(q1) - xD*sin(q1)), 0, 0 ; ...
       0, l1*(2*dr*sin(q2) + 2*zD*cos(q2) + xD*sin(q2) - 3^(1/2)*yD*sin(q2)), 0; ...
       0, 0, l1*(2*dr*sin(q3) + 2*zD*cos(q3) + xD*sin(q3) + 3^(1/2)*yD*sin(q3))];
end

function [dJc,dJq] = dJcq(xD,yD,zD,dxD,dyD,dzD,dr,l1,q1,q2,q3,dq1,dq2,dq3)
dJc = [2*dxD + 2*l1*sin(q1)*dq1, 2*dyD, 2*dzD - 2*l1*cos(q1)*dq1 ; ...
       2*dxD - l1*sin(q2)*dq2, 2*dyD + 3^(1/2)*l1*sin(q2)*dq2, 2*dzD - 2*l1*cos(q2)*dq2 ; ...
       2*dxD - l1*sin(q3)*dq3, 2*dyD - 3^(1/2)*l1*sin(q3)*dq3, 2*dzD - 2*l1*cos(q3)*dq3];
dJq = [-2*l1*(sin(q1)*dxD - cos(q1)*dzD + cos(q1)*xD*dq1 + sin(q1)*zD*dq1 - dr*cos(q1)*dq1), 0, 0 ; ...
        0, l1*(2*cos(q2)*dzD + sin(q2)*dxD + cos(q2)*xD*dq2 - 2*sin(q2)*zD*dq2 + 2*dr*cos(q2)*dq2 - 3^(1/2)*sin(q2)*dyD - 3^(1/2)*cos(q2)*yD*dq2), 0 ; ...
        0, 0, l1*(2*cos(q3)*dzD + sin(q3)*dxD + cos(q3)*xD*dq3 - 2*sin(q3)*zD*dq3 + 2*dr*cos(q3)*dq3 + 3^(1/2)*sin(q3)*dyD + 3^(1/2)*cos(q3)*yD*dq3)];
end

function [c11,c21,c31,c12,c22,c32] = f_cii(r4,x,q4,q5) 
r45 = r4 + x*sin(q5);
% The derivatives below are obtained wrt D = H - t_r
c11 = r45*sin(q4); 
c21 = -r45*cos(q4);
c31 = 0;
c12 = -x*cos(q4)*cos(q5);
c22 = -x*sin(q4)*cos(q5);
c32 = -x*sin(q5);
end

function [dc11,dc21,dc31,dc12,dc22,dc32] = f_deriv_cii(r4,x,q4,q5,dq4,dq5) 
r45 = r4 + x*sin(q5);

dc11 = x*cos(q5)*sin(q4)*dq5 + r45*cos(q4)*dq4;
dc21 = -x*cos(q5)*cos(q4)*dq5 + r45*sin(q4)*dq4;
dc31 = 0;
dc12 = x*sin(q4)*cos(q5)*dq4 + x*cos(q4)*sin(q5)*dq5;
dc22 = -x*cos(q4)*cos(q5)*dq4 + x*sin(q4)*sin(q5)*dq5;
dc32 = -x*cos(q5)*dq5;
end

function [c11F,c21F,c31F,dc11F,dc21F,dc31F] = f_d_ciiF(x,q4,dq4)
c11F = x*sin(q4); 
c21F = -x*cos(q4);
c31F = 0;
dc11F = x*cos(q4)*dq4; 
dc21F = x*sin(q4)*dq4;
dc31F = 0;
end

== matlab function RL5_6kg_2021a_enc/AXIS Scopes & Reorganization of outputs/TCP comparison D and H/D-H verification ==
  data: Dpos input; q45 input; Hpos_c output
function Hpos_c = jacob(Dpos,q45)

r4 =  0.0632;   % [m], radius of wrist arm offset, distance from point E to F
h4 =  0.132;    % [m], perpendicular distance from point D to E
r5 =  0.135;    % [m], radius of swivel arm (distance A5-axis vs. Tool Center Point (TCP))

% Wrist arm joint positions
q4 = q45(1);
q5 = q45(2);

% Point D position 
xD = Dpos(1);
yD = Dpos(2);
zD = Dpos(3);

% Eq (8) in the paper
xH = xD + cos(q4)*(r4 + r5*sin(q5));
yH = yD + sin(q4)*(r4 + r5*sin(q5));
zH = zD - h4 - r5*cos(q5); 

Hpos_c = [xH; yH; zH];      % Calculated Point H position

== matlab function RL5_6kg_2021a_enc/Kinematic model ==
  data: dD input; D input; q input; dq input; dH_c output; ddq input; ddH_c output
function [dH_c, ddH_c] = kin(dD,D,q,dq,ddq)
% This function block represents FORWARD KINEMATICS FOR VELOCITY 

q0 = 5.327998*pi/180;   % [rad], 5.327998° ~ q0*pi/180 rad, angle( axis_i & line(A_i,B_i) )
r0 =  0.330;            % [m], radius of circumscribed circle of equilat. basic frame triangle
l1 =  0.420;            % [m], lengths of upper arms
% l2 =  1.055;          % [m], lengths of forearms, not used
r3 =  0.125;            % [m], radius of circumscribed circle of equilat. mov. platform trngl.
r4 =  0.0632;           % [m], radius of wrist arm offset, distance from point E to F
% h4 =  0.132;          % [m], perpendicular distance from point D to E (h4m = h4), not used
r5 =  0.135;            % [m], radius of swivel arm (distance A5-axis vs. Tool Center Point (TCP)), not used
dr =  r0 - r3;          % [m], useful simplifying constant

% Actuated joint positions
q1 = q(1) - q0; q2 = q(2) - q0;  q3 = q(3) - q0;  q4 = q(4);  q5 = q(5);

% Actuated joint velocities
dq1 = dq(1);  dq2 = dq(2);  dq3 = dq(3);  dq4 = dq(4);  dq5 = dq(5);

% Actuated joint accelerations
% ddq1 = ddq(1);  ddq2 = ddq(2);  ddq3 = ddq(3);  ddq4 = ddq(4);  ddq5 = ddq(5);

% Point D position
xD = D(1);  yD = D(2);  zD = D(3); 

% Point D velocity
dxD = dD(1);  dyD = dD(2);  dzD = dD(3);

%% Jacobian matrices J_D, J_q, J_\mathcal{D}, J and their derivatives and inverses

[Jd,Jq] = Jcq(xD,yD,zD,dr,l1,q1,q2,q3);             % Eq (17) in the paper: Jd = J_D, Jq = J_q 
Jqd = Jd\Jq; iJqd = Jq\Jd;                          % Eq (18) in the paper: Jqd = J_qD, iJqd = J_qD^{-1}

JD = [Jqd, zeros(3,2); zeros(2,3), eye(2)];         % Eq (19) in the paper: JD = J_\mathcal{D}
% iJD = [iJqd, zeros(3,2) ; zeros(2,3), eye(2)];    % Eq (19) in the paper: iJD = J_\mathcal{D}^{-1}, not used

[dJc,dJq] = dJcq(xD,yD,zD,dxD,dyD,dzD,dr,l1,q1,q2,q3,dq1,dq2,dq3); 
dJqd = Jd\(dJq-dJc*Jqd);                            % Eq (22) in the paper: derivative of J_qD

dJD = [dJqd, zeros(3,2) ; zeros(2,3), zeros(2)];    % derivative of J_\mathcal{D}

[c11,c21,c31,c12,c22,c32] = f_cii(r4,r5,q4,q5);    
Jsc = [c11, c12 ; c21, c22 ; c31, c32]; 
iJDH = [eye(3), Jsc ; zeros(2,3), eye(2)];          % Eq (15) in the paper: iJDH = J_\mathcal{DH}^{-1}

J = iJDH\JD;                                        % Eq (26) with (19) in the paper: J_\mathcal{H} = J_\mathcal{DH}^{-1}*J_\mathcal{D}

[dc11,dc21,dc31,dc12,dc22,dc32] = f_deriv_cii(r4,r5,q4,q5,dq4,dq5); 
dJsc = [dc11, dc12 ; dc21, dc22 ; dc31, dc32]; 
diJDH = [zeros(3), dJsc ; zeros(2,3), zeros(2)];    % derivative of J_\mathcal{DH}

dJ = (iJDH\(dJD - diJDH*J));                        % derivative of J_\mathcal{H}


%% Calculated point H velocity and acceleration
dH_c = J*dq;               % Eq. (19) in the paper
ddH_c = dJ*dq + J*ddq ;    % Eq. (23) in the paper

end

function [Jc,Jq] = Jcq(xD,yD,zD,dr,l1,q1,q2,q3)
Jc = [ 2*xD - 2*dr - 2*l1*cos(q1),                                   2*yD, 2*zD - 2*l1*sin(q1); ...
       dr + 2*xD + l1*cos(q2), 2*yD - 3^(1/2)*dr - 3^(1/2)*l1*cos(q2), 2*zD - 2*l1*sin(q2); ...
       dr + 2*xD + l1*cos(q3), 2*yD + 3^(1/2)*dr + 3^(1/2)*l1*cos(q3), 2*zD - 2*l1*sin(q3)];
Jq = [ 2*l1*(dr*sin(q1) + zD*cos(q1) - xD*sin(q1)), 0, 0 ; ...
       0, l1*(2*dr*sin(q2) + 2*zD*cos(q2) + xD*sin(q2) - 3^(1/2)*yD*sin(q2)), 0; ...
       0, 0, l1*(2*dr*sin(q3) + 2*zD*cos(q3) + xD*sin(q3) + 3^(1/2)*yD*sin(q3))];
end

function [dJc,dJq] = dJcq(xD,yD,zD,dxD,dyD,dzD,dr,l1,q1,q2,q3,dq1,dq2,dq3)
dJc = [2*dxD + 2*l1*sin(q1)*dq1, 2*dyD, 2*dzD - 2*l1*cos(q1)*dq1 ; ...
       2*dxD - l1*sin(q2)*dq2, 2*dyD + 3^(1/2)*l1*sin(q2)*dq2, 2*dzD - 2*l1*cos(q2)*dq2 ; ...
       2*dxD - l1*sin(q3)*dq3, 2*dyD - 3^(1/2)*l1*sin(q3)*dq3, 2*dzD - 2*l1*cos(q3)*dq3];
dJq = [-2*l1*(sin(q1)*dxD - cos(q1)*dzD + cos(q1)*xD*dq1 + sin(q1)*zD*dq1 - dr*cos(q1)*dq1), 0, 0 ; ...
        0, l1*(2*cos(q2)*dzD + sin(q2)*dxD + cos(q2)*xD*dq2 - 2*sin(q2)*zD*dq2 + 2*dr*cos(q2)*dq2 - 3^(1/2)*sin(q2)*dyD - 3^(1/2)*cos(q2)*yD*dq2), 0 ; ...
        0, 0, l1*(2*cos(q3)*dzD + sin(q3)*dxD + cos(q3)*xD*dq3 - 2*sin(q3)*zD*dq3 + 2*dr*cos(q3)*dq3 + 3^(1/2)*sin(q3)*dyD + 3^(1/2)*cos(q3)*yD*dq3)];
end

function [c11,c21,c31,c12,c22,c32] = f_cii(r4,x,q4,q5) % x will stand for lH, r4m, r5m
r45 = r4 + x*sin(q5);
% The derivatives below are obtained wrt D = H - t_r
c11 = r45*sin(q4); 
c21 = -r45*cos(q4);
c31 = 0;
c12 = -x*cos(q4)*cos(q5);
c22 = -x*sin(q4)*cos(q5);
c32 = -x*sin(q5);
end

function [dc11,dc21,dc31,dc12,dc22,dc32] = f_deriv_cii(r4,x,q4,q5,dq4,dq5) % x will stand for lH, r4m, r5m
r45 = r4 + x*sin(q5);

dc11 = x*cos(q5)*sin(q4)*dq5 + r45*cos(q4)*dq4;
dc21 = -x*cos(q5)*cos(q4)*dq5 + r45*sin(q4)*dq4;
dc31 = 0;
dc12 = x*sin(q4)*cos(q5)*dq4 + x*cos(q4)*sin(q5)*dq5;
dc22 = -x*cos(q4)*cos(q5)*dq4 + x*sin(q4)*sin(q5)*dq5;
dc32 = -x*cos(q5)*dq5;
end

function [c11F,c21F,c31F,dc11F,dc21F,dc31F] = f_d_ciiF(x,q4,dq4)
c11F = x*sin(q4); 
c21F = -x*cos(q4);
c31F = 0;
dc11F = x*cos(q4)*dq4; 
dc21F = x*sin(q4)*dq4;
dc31F = 0;
end
